simulink model "namrata_lab7_2"  (R2018b)
settings: Solver=VariableStepAuto  StartTime=0.0  StopTime=10.0  RelTol=1e-3
settings Model: Creator=student  LastModifiedBy=student

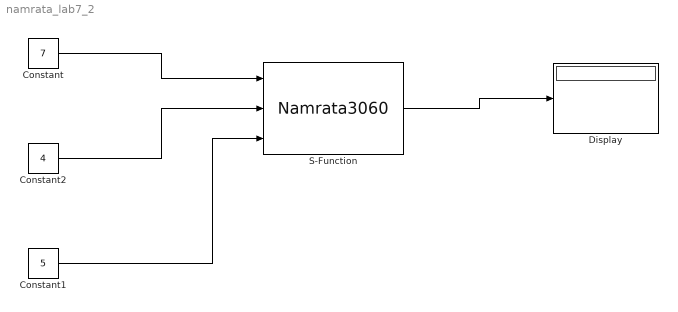
== system namrata_lab7_2 ==
  Constant : Constant  Value=7
  Constant1 : Constant  Value=5
  Constant2 : Constant  Value=4
  Display : Display
  S-Function : S-Function  FunctionName=Namrata3060  SFunctionDeploymentMode=off  EnableBusSupport=off
  wires:
  Constant/1 -> S-Function/1
  Constant2/1 -> S-Function/2
  S-Function/1 -> Display/1
  Constant1/1 -> S-Function/3
